simulink subsystem "Reductor2"  (R2023a)
settings: Solver=VariableStepAuto  StartTime=0.0  StopTime=10.0  RelTol=1e-3
model mask{J=0, i=0}
  mask prompts: J "Reductor inertia"; i "Reductor ratio"
settings Model: Creator=ycheb  LastModifiedBy=ycheb

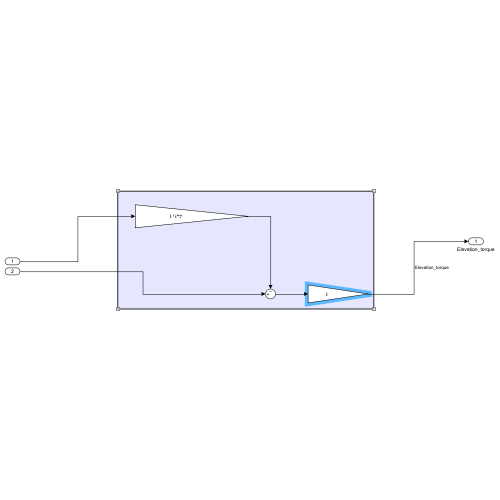
[thumbnail: Simulink's stored preview of the top-level diagram]
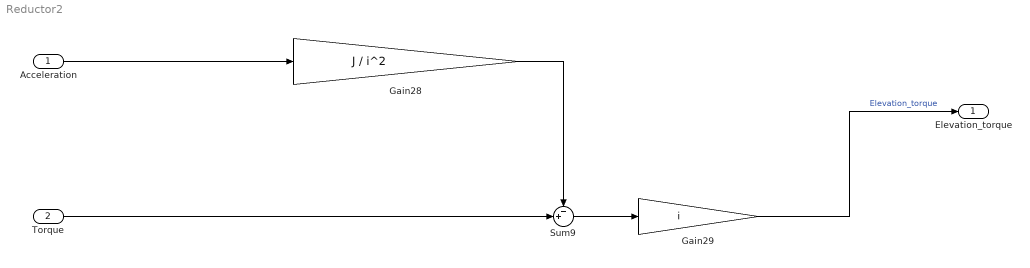
== system Reductor2 ==
  Acceleration : Inport
  Torque : Inport  Port=2
  Gain28 : Gain  Gain=J / i^2
  Gain29 : Gain  Gain=i
  Sum9 : Sum  Inputs=-+|
  Elevation_torque : Outport
  wires:
  Gain28/1 -> Sum9/1
  Gain29/1 -> Elevation_torque/1  "Elevation_torque"
  Torque/1 -> Sum9/2
  Acceleration/1 -> Gain28/1
  Sum9/1 -> Gain29/1
